simulink subsystem "ALU_64_BITS_05_SS"  (R2022a)
settings: Solver=VariableStepAuto  StartTime=0.0  StopTime=10.0  RelTol=1e-3
libraries: hdlBasic x1540
(part 1 of 7)
settings Model: Creator=sebas  LastModifiedBy=viktor

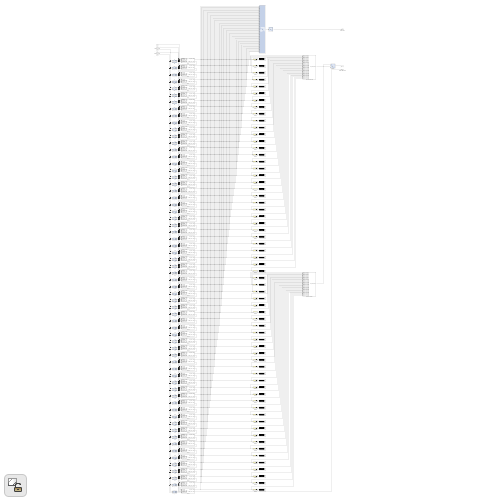
[thumbnail: Simulink's stored preview of the top-level diagram]
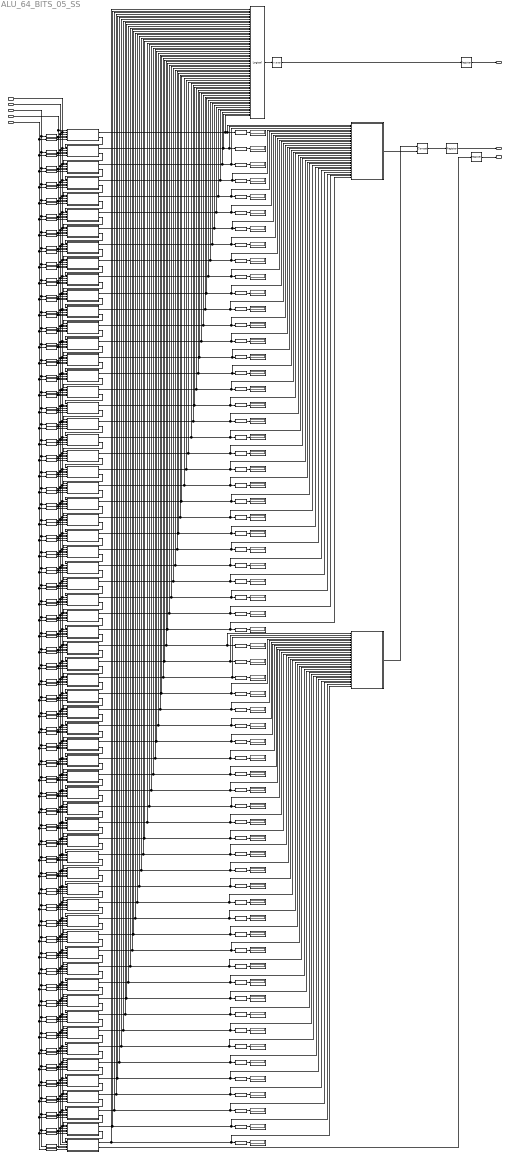
== system ALU_64_BITS_05_SS ==
  OPERATION (2 BIT) : Inport
  A_INVERT (1 BIT) : Inport  Port=2
  A_INPUT (64 BIT) : Inport  Port=3
  B_INVERT (1 BIT) : Inport  Port=4
  B_INPUT (64 BIT) : Inport  Port=5
  ALU_0 : Subsystem
  ALU_1 : Subsystem
  ALU_10 : Subsystem
  ALU_11 : Subsystem
  ALU_12 : Subsystem
  ALU_13 : Subsystem
  ALU_14 : Subsystem
  ALU_15 : Subsystem
  ALU_16 : Subsystem
  ALU_17 : Subsystem
  ALU_18 : Subsystem
  ALU_19 : Subsystem
  ALU_2 : Subsystem
  ALU_20 : Subsystem
  ALU_21 : Subsystem
  ALU_22 : Subsystem
  ALU_23 : Subsystem
  ALU_24 : Subsystem
  ALU_25 : Subsystem
  ALU_26 : Subsystem
  ALU_27 : Subsystem
  ALU_28 : Subsystem
  ALU_29 : Subsystem
  ALU_3 : Subsystem
  ALU_30 : Subsystem
  ALU_31 : Subsystem
  ALU_32 : Subsystem
  ALU_33 : Subsystem
  ALU_34 : Subsystem
  ALU_35 : Subsystem
  ALU_36 : Subsystem
  ALU_37 : Subsystem
  ALU_38 : Subsystem
  ALU_39 : Subsystem
  ALU_4 : Subsystem
  ALU_40 : Subsystem
  ALU_41 : Subsystem
  ALU_42 : Subsystem
  ALU_43 : Subsystem
  ALU_44 : Subsystem
  ALU_45 : Subsystem
  ALU_46 : Subsystem
  ALU_47 : Subsystem
  ALU_48 : Subsystem
  ALU_49 : Subsystem
  ALU_5 : Subsystem
  ALU_50 : Subsystem
  ALU_51 : Subsystem
  ALU_52 : Subsystem
  ALU_53 : Subsystem
  ALU_54 : Subsystem
  ALU_55 : Subsystem
  ALU_56 : Subsystem
  ALU_57 : Subsystem
  ALU_58 : Subsystem
  ALU_59 : Subsystem
  ALU_6 : Subsystem
  ALU_60 : Subsystem
  ALU_61 : Subsystem
  ALU_62 : Subsystem
  ALU_63 : Subsystem
  ALU_7 : Subsystem
  ALU_8 : Subsystem
  ALU_9 : Subsystem
  ALU_OUT_32_BIT_00 : Subsystem
  ALU_OUT_32_BIT_1 : Subsystem
  A_0 : hdlBasic/Slice  nbits=1  boolean_output=off  mode=Lower Bit Location + Width  bit1=-3  base1=MSB of Input  bit0=0  base0=LSB of Input  XmcBlockStatus=1  maskContainerNames=group1  block_type=slice  block_config=sysgen:Slice_config
  A_1 : hdlBasic/Slice  nbits=1  boolean_output=off  mode=Lower Bit Location + Width  bit1=-3  base1=MSB of Input  bit0=1  base0=LSB of Input  XmcBlockStatus=1  maskContainerNames=group1  block_type=slice  block_config=sysgen:Slice_config
  A_10 : hdlBasic/Slice  nbits=1  boolean_output=off  mode=Lower Bit Location + Width  bit1=-3  base1=MSB of Input  bit0=10  base0=LSB of Input  XmcBlockStatus=1  maskContainerNames=group1  block_type=slice  block_config=sysgen:Slice_config
  A_11 : hdlBasic/Slice  nbits=1  boolean_output=off  mode=Lower Bit Location + Width  bit1=-3  base1=MSB of Input  bit0=11  base0=LSB of Input  XmcBlockStatus=1  maskContainerNames=group1  block_type=slice  block_config=sysgen:Slice_config
  A_12 : hdlBasic/Slice  nbits=1  boolean_output=off  mode=Lower Bit Location + Width  bit1=-3  base1=MSB of Input  bit0=12  base0=LSB of Input  XmcBlockStatus=1  maskContainerNames=group1  block_type=slice  block_config=sysgen:Slice_config
  A_13 : hdlBasic/Slice  nbits=1  boolean_output=off  mode=Lower Bit Location + Width  bit1=-3  base1=MSB of Input  bit0=13  base0=LSB of Input  XmcBlockStatus=1  maskContainerNames=group1  block_type=slice  block_config=sysgen:Slice_config
  A_14 : hdlBasic/Slice  nbits=1  boolean_output=off  mode=Lower Bit Location + Width  bit1=-3  base1=MSB of Input  bit0=14  base0=LSB of Input  XmcBlockStatus=1  maskContainerNames=group1  block_type=slice  block_config=sysgen:Slice_config
  A_15 : hdlBasic/Slice  nbits=1  boolean_output=off  mode=Lower Bit Location + Width  bit1=-3  base1=MSB of Input  bit0=15  base0=LSB of Input  XmcBlockStatus=1  maskContainerNames=group1  block_type=slice  block_config=sysgen:Slice_config
  A_16 : hdlBasic/Slice  nbits=1  boolean_output=off  mode=Lower Bit Location + Width  bit1=-3  base1=MSB of Input  bit0=16  base0=LSB of Input  XmcBlockStatus=1  maskContainerNames=group1  block_type=slice  block_config=sysgen:Slice_config
  A_17 : hdlBasic/Slice  nbits=1  boolean_output=off  mode=Lower Bit Location + Width  bit1=-3  base1=MSB of Input  bit0=17  base0=LSB of Input  XmcBlockStatus=1  maskContainerNames=group1  block_type=slice  block_config=sysgen:Slice_config
  A_18 : hdlBasic/Slice  nbits=1  boolean_output=off  mode=Lower Bit Location + Width  bit1=-3  base1=MSB of Input  bit0=18  base0=LSB of Input  XmcBlockStatus=1  maskContainerNames=group1  block_type=slice  block_config=sysgen:Slice_config
  A_19 : hdlBasic/Slice  nbits=1  boolean_output=off  mode=Lower Bit Location + Width  bit1=-3  base1=MSB of Input  bit0=19  base0=LSB of Input  XmcBlockStatus=1  maskContainerNames=group1  block_type=slice  block_config=sysgen:Slice_config
  A_2 : hdlBasic/Slice  nbits=1  boolean_output=off  mode=Lower Bit Location + Width  bit1=-3  base1=MSB of Input  bit0=2  base0=LSB of Input  XmcBlockStatus=1  maskContainerNames=group1  block_type=slice  block_config=sysgen:Slice_config
  A_20 : hdlBasic/Slice  nbits=1  boolean_output=off  mode=Lower Bit Location + Width  bit1=-3  base1=MSB of Input  bit0=20  base0=LSB of Input  XmcBlockStatus=1  maskContainerNames=group1  block_type=slice  block_config=sysgen:Slice_config
  A_21 : hdlBasic/Slice  nbits=1  boolean_output=off  mode=Lower Bit Location + Width  bit1=-3  base1=MSB of Input  bit0=21  base0=LSB of Input  XmcBlockStatus=1  maskContainerNames=group1  block_type=slice  block_config=sysgen:Slice_config
  A_22 : hdlBasic/Slice  nbits=1  boolean_output=off  mode=Lower Bit Location + Width  bit1=-3  base1=MSB of Input  bit0=22  base0=LSB of Input  XmcBlockStatus=1  maskContainerNames=group1  block_type=slice  block_config=sysgen:Slice_config
  A_23 : hdlBasic/Slice  nbits=1  boolean_output=off  mode=Lower Bit Location + Width  bit1=-3  base1=MSB of Input  bit0=23  base0=LSB of Input  XmcBlockStatus=1  maskContainerNames=group1  block_type=slice  block_config=sysgen:Slice_config
  A_24 : hdlBasic/Slice  nbits=1  boolean_output=off  mode=Lower Bit Location + Width  bit1=-3  base1=MSB of Input  bit0=24  base0=LSB of Input  XmcBlockStatus=1  maskContainerNames=group1  block_type=slice  block_config=sysgen:Slice_config
  A_25 : hdlBasic/Slice  nbits=1  boolean_output=off  mode=Lower Bit Location + Width  bit1=-3  base1=MSB of Input  bit0=25  base0=LSB of Input  XmcBlockStatus=1  maskContainerNames=group1  block_type=slice  block_config=sysgen:Slice_config
  A_26 : hdlBasic/Slice  nbits=1  boolean_output=off  mode=Lower Bit Location + Width  bit1=-3  base1=MSB of Input  bit0=26  base0=LSB of Input  XmcBlockStatus=1  maskContainerNames=group1  block_type=slice  block_config=sysgen:Slice_config
  A_27 : hdlBasic/Slice  nbits=1  boolean_output=off  mode=Lower Bit Location + Width  bit1=-3  base1=MSB of Input  bit0=27  base0=LSB of Input  XmcBlockStatus=1  maskContainerNames=group1  block_type=slice  block_config=sysgen:Slice_config
  A_28 : hdlBasic/Slice  nbits=1  boolean_output=off  mode=Lower Bit Location + Width  bit1=-3  base1=MSB of Input  bit0=28  base0=LSB of Input  XmcBlockStatus=1  maskContainerNames=group1  block_type=slice  block_config=sysgen:Slice_config
  A_29 : hdlBasic/Slice  nbits=1  boolean_output=off  mode=Lower Bit Location + Width  bit1=-3  base1=MSB of Input  bit0=29  base0=LSB of Input  XmcBlockStatus=1  maskContainerNames=group1  block_type=slice  block_config=sysgen:Slice_config
  A_3 : hdlBasic/Slice  nbits=1  boolean_output=off  mode=Lower Bit Location + Width  bit1=-3  base1=MSB of Input  bit0=3  base0=LSB of Input  XmcBlockStatus=1  maskContainerNames=group1  block_type=slice  block_config=sysgen:Slice_config
  A_30 : hdlBasic/Slice  nbits=1  boolean_output=off  mode=Lower Bit Location + Width  bit1=-3  base1=MSB of Input  bit0=30  base0=LSB of Input  XmcBlockStatus=1  maskContainerNames=group1  block_type=slice  block_config=sysgen:Slice_config
  A_31 : hdlBasic/Slice  nbits=1  boolean_output=off  mode=Lower Bit Location + Width  bit1=-3  base1=MSB of Input  bit0=31  base0=LSB of Input  XmcBlockStatus=1  maskContainerNames=group1  block_type=slice  block_config=sysgen:Slice_config
  A_32 : hdlBasic/Slice  nbits=1  boolean_output=off  mode=Lower Bit Location + Width  bit1=-3  base1=MSB of Input  bit0=32  base0=LSB of Input  XmcBlockStatus=1  maskContainerNames=group1  block_type=slice  block_config=sysgen:Slice_config
  A_33 : hdlBasic/Slice  nbits=1  boolean_output=off  mode=Lower Bit Location + Width  bit1=-3  base1=MSB of Input  bit0=33  base0=LSB of Input  XmcBlockStatus=1  maskContainerNames=group1  block_type=slice  block_config=sysgen:Slice_config
  A_34 : hdlBasic/Slice  nbits=1  boolean_output=off  mode=Lower Bit Location + Width  bit1=-3  base1=MSB of Input  bit0=34  base0=LSB of Input  XmcBlockStatus=1  maskContainerNames=group1  block_type=slice  block_config=sysgen:Slice_config
  A_35 : hdlBasic/Slice  nbits=1  boolean_output=off  mode=Lower Bit Location + Width  bit1=-3  base1=MSB of Input  bit0=35  base0=LSB of Input  XmcBlockStatus=1  maskContainerNames=group1  block_type=slice  block_config=sysgen:Slice_config
  A_36 : hdlBasic/Slice  nbits=1  boolean_output=off  mode=Lower Bit Location + Width  bit1=-3  base1=MSB of Input  bit0=36  base0=LSB of Input  XmcBlockStatus=1  maskContainerNames=group1  block_type=slice  block_config=sysgen:Slice_config
  A_37 : hdlBasic/Slice  nbits=1  boolean_output=off  mode=Lower Bit Location + Width  bit1=-3  base1=MSB of Input  bit0=37  base0=LSB of Input  XmcBlockStatus=1  maskContainerNames=group1  block_type=slice  block_config=sysgen:Slice_config
  A_38 : hdlBasic/Slice  nbits=1  boolean_output=off  mode=Lower Bit Location + Width  bit1=-3  base1=MSB of Input  bit0=38  base0=LSB of Input  XmcBlockStatus=1  maskContainerNames=group1  block_type=slice  block_config=sysgen:Slice_config
  A_39 : hdlBasic/Slice  nbits=1  boolean_output=off  mode=Lower Bit Location + Width  bit1=-3  base1=MSB of Input  bit0=39  base0=LSB of Input  XmcBlockStatus=1  maskContainerNames=group1  block_type=slice  block_config=sysgen:Slice_config
  A_4 : hdlBasic/Slice  nbits=1  boolean_output=off  mode=Lower Bit Location + Width  bit1=-3  base1=MSB of Input  bit0=4  base0=LSB of Input  XmcBlockStatus=1  maskContainerNames=group1  block_type=slice  block_config=sysgen:Slice_config
  A_40 : hdlBasic/Slice  nbits=1  boolean_output=off  mode=Lower Bit Location + Width  bit1=-3  base1=MSB of Input  bit0=40  base0=LSB of Input  XmcBlockStatus=1  maskContainerNames=group1  block_type=slice  block_config=sysgen:Slice_config
  A_41 : hdlBasic/Slice  nbits=1  boolean_output=off  mode=Lower Bit Location + Width  bit1=-3  base1=MSB of Input  bit0=41  base0=LSB of Input  XmcBlockStatus=1  maskContainerNames=group1  block_type=slice  block_config=sysgen:Slice_config
  A_42 : hdlBasic/Slice  nbits=1  boolean_output=off  mode=Lower Bit Location + Width  bit1=-3  base1=MSB of Input  bit0=42  base0=LSB of Input  XmcBlockStatus=1  maskContainerNames=group1  block_type=slice  block_config=sysgen:Slice_config
  A_43 : hdlBasic/Slice  nbits=1  boolean_output=off  mode=Lower Bit Location + Width  bit1=-3  base1=MSB of Input  bit0=43  base0=LSB of Input  XmcBlockStatus=1  maskContainerNames=group1  block_type=slice  block_config=sysgen:Slice_config
  A_44 : hdlBasic/Slice  nbits=1  boolean_output=off  mode=Lower Bit Location + Width  bit1=-3  base1=MSB of Input  bit0=44  base0=LSB of Input  XmcBlockStatus=1  maskContainerNames=group1  block_type=slice  block_config=sysgen:Slice_config
  A_45 : hdlBasic/Slice  nbits=1  boolean_output=off  mode=Lower Bit Location + Width  bit1=-3  base1=MSB of Input  bit0=45  base0=LSB of Input  XmcBlockStatus=1  maskContainerNames=group1  block_type=slice  block_config=sysgen:Slice_config
  A_46 : hdlBasic/Slice  nbits=1  boolean_output=off  mode=Lower Bit Location + Width  bit1=-3  base1=MSB of Input  bit0=46  base0=LSB of Input  XmcBlockStatus=1  maskContainerNames=group1  block_type=slice  block_config=sysgen:Slice_config
  A_47 : hdlBasic/Slice  nbits=1  boolean_output=off  mode=Lower Bit Location + Width  bit1=-3  base1=MSB of Input  bit0=47  base0=LSB of Input  XmcBlockStatus=1  maskContainerNames=group1  block_type=slice  block_config=sysgen:Slice_config
  A_48 : hdlBasic/Slice  nbits=1  boolean_output=off  mode=Lower Bit Location + Width  bit1=-3  base1=MSB of Input  bit0=48  base0=LSB of Input  XmcBlockStatus=1  maskContainerNames=group1  block_type=slice  block_config=sysgen:Slice_config
  A_49 : hdlBasic/Slice  nbits=1  boolean_output=off  mode=Lower Bit Location + Width  bit1=-3  base1=MSB of Input  bit0=49  base0=LSB of Input  XmcBlockStatus=1  maskContainerNames=group1  block_type=slice  block_config=sysgen:Slice_config
  A_5 : hdlBasic/Slice  nbits=1  boolean_output=off  mode=Lower Bit Location + Width  bit1=-3  base1=MSB of Input  bit0=5  base0=LSB of Input  XmcBlockStatus=1  maskContainerNames=group1  block_type=slice  block_config=sysgen:Slice_config
  A_50 : hdlBasic/Slice  nbits=1  boolean_output=off  mode=Lower Bit Location + Width  bit1=-3  base1=MSB of Input  bit0=50  base0=LSB of Input  XmcBlockStatus=1  maskContainerNames=group1  block_type=slice  block_config=sysgen:Slice_config
  A_51 : hdlBasic/Slice  nbits=1  boolean_output=off  mode=Lower Bit Location + Width  bit1=-3  base1=MSB of Input  bit0=51  base0=LSB of Input  XmcBlockStatus=1  maskContainerNames=group1  block_type=slice  block_config=sysgen:Slice_config
  A_52 : hdlBasic/Slice  nbits=1  boolean_output=off  mode=Lower Bit Location + Width  bit1=-3  base1=MSB of Input  bit0=52  base0=LSB of Input  XmcBlockStatus=1  maskContainerNames=group1  block_type=slice  block_config=sysgen:Slice_config
  A_53 : hdlBasic/Slice  nbits=1  boolean_output=off  mode=Lower Bit Location + Width  bit1=-3  base1=MSB of Input  bit0=53  base0=LSB of Input  XmcBlockStatus=1  maskContainerNames=group1  block_type=slice  block_config=sysgen:Slice_config
  A_54 : hdlBasic/Slice  nbits=1  boolean_output=off  mode=Lower Bit Location + Width  bit1=-3  base1=MSB of Input  bit0=54  base0=LSB of Input  XmcBlockStatus=1  maskContainerNames=group1  block_type=slice  block_config=sysgen:Slice_config
  A_55 : hdlBasic/Slice  nbits=1  boolean_output=off  mode=Lower Bit Location + Width  bit1=-3  base1=MSB of Input  bit0=55  base0=LSB of Input  XmcBlockStatus=1  maskContainerNames=group1  block_type=slice  block_config=sysgen:Slice_config
  A_56 : hdlBasic/Slice  nbits=1  boolean_output=off  mode=Lower Bit Location + Width  bit1=-3  base1=MSB of Input  bit0=56  base0=LSB of Input  XmcBlockStatus=1  maskContainerNames=group1  block_type=slice  block_config=sysgen:Slice_config
  A_57 : hdlBasic/Slice  nbits=1  boolean_output=off  mode=Lower Bit Location + Width  bit1=-3  base1=MSB of Input  bit0=57  base0=LSB of Input  XmcBlockStatus=1  maskContainerNames=group1  block_type=slice  block_config=sysgen:Slice_config
  A_58 : hdlBasic/Slice  nbits=1  boolean_output=off  mode=Lower Bit Location + Width  bit1=-3  base1=MSB of Input  bit0=58  base0=LSB of Input  XmcBlockStatus=1  maskContainerNames=group1  block_type=slice  block_config=sysgen:Slice_config
  A_59 : hdlBasic/Slice  nbits=1  boolean_output=off  mode=Lower Bit Location + Width  bit1=-3  base1=MSB of Input  bit0=59  base0=LSB of Input  XmcBlockStatus=1  maskContainerNames=group1  block_type=slice  block_config=sysgen:Slice_config
  A_6 : hdlBasic/Slice  nbits=1  boolean_output=off  mode=Lower Bit Location + Width  bit1=-3  base1=MSB of Input  bit0=6  base0=LSB of Input  XmcBlockStatus=1  maskContainerNames=group1  block_type=slice  block_config=sysgen:Slice_config
  A_60 : hdlBasic/Slice  nbits=1  boolean_output=off  mode=Lower Bit Location + Width  bit1=-3  base1=MSB of Input  bit0=60  base0=LSB of Input  XmcBlockStatus=1  maskContainerNames=group1  block_type=slice  block_config=sysgen:Slice_config
  A_61 : hdlBasic/Slice  nbits=1  boolean_output=off  mode=Lower Bit Location + Width  bit1=-3  base1=MSB of Input  bit0=61  base0=LSB of Input  XmcBlockStatus=1  maskContainerNames=group1  block_type=slice  block_config=sysgen:Slice_config
  A_62 : hdlBasic/Slice  nbits=1  boolean_output=off  mode=Lower Bit Location + Width  bit1=-3  base1=MSB of Input  bit0=62  base0=LSB of Input  XmcBlockStatus=1  maskContainerNames=group1  block_type=slice  block_config=sysgen:Slice_config
  A_63 : hdlBasic/Slice  nbits=1  boolean_output=off  mode=Lower Bit Location + Width  bit1=-3  base1=MSB of Input  bit0=63  base0=LSB of Input  XmcBlockStatus=1  maskContainerNames=group1  block_type=slice  block_config=sysgen:Slice_config
  A_7 : hdlBasic/Slice  nbits=1  boolean_output=off  mode=Lower Bit Location + Width  bit1=-3  base1=MSB of Input  bit0=7  base0=LSB of Input  XmcBlockStatus=1  maskContainerNames=group1  block_type=slice  block_config=sysgen:Slice_config
  A_8 : hdlBasic/Slice  nbits=1  boolean_output=off  mode=Lower Bit Location + Width  bit1=-3  base1=MSB of Input  bit0=8  base0=LSB of Input  XmcBlockStatus=1  maskContainerNames=group1  block_type=slice  block_config=sysgen:Slice_config
  A_9 : hdlBasic/Slice  nbits=1  boolean_output=off  mode=Lower Bit Location + Width  bit1=-3  base1=MSB of Input  bit0=9  base0=LSB of Input  XmcBlockStatus=1  maskContainerNames=group1  block_type=slice  block_config=sysgen:Slice_config
  B_0 : hdlBasic/Slice  nbits=1  boolean_output=off  mode=Lower Bit Location + Width  bit1=-3  base1=MSB of Input  bit0=0  base0=LSB of Input  XmcBlockStatus=1  maskContainerNames=group1  block_type=slice  block_config=sysgen:Slice_config
  B_1 : hdlBasic/Slice  nbits=1  boolean_output=off  mode=Lower Bit Location + Width  bit1=-3  base1=MSB of Input  bit0=1  base0=LSB of Input  XmcBlockStatus=1  maskContainerNames=group1  block_type=slice  block_config=sysgen:Slice_config
  B_10 : hdlBasic/Slice  nbits=1  boolean_output=off  mode=Lower Bit Location + Width  bit1=-3  base1=MSB of Input  bit0=10  base0=LSB of Input  XmcBlockStatus=1  maskContainerNames=group1  block_type=slice  block_config=sysgen:Slice_config
  B_11 : hdlBasic/Slice  nbits=1  boolean_output=off  mode=Lower Bit Location + Width  bit1=-3  base1=MSB of Input  bit0=11  base0=LSB of Input  XmcBlockStatus=1  maskContainerNames=group1  block_type=slice  block_config=sysgen:Slice_config
  B_12 : hdlBasic/Slice  nbits=1  boolean_output=off  mode=Lower Bit Location + Width  bit1=-3  base1=MSB of Input  bit0=12  base0=LSB of Input  XmcBlockStatus=1  maskContainerNames=group1  block_type=slice  block_config=sysgen:Slice_config
  B_13 : hdlBasic/Slice  nbits=1  boolean_output=off  mode=Lower Bit Location + Width  bit1=-3  base1=MSB of Input  bit0=13  base0=LSB of Input  XmcBlockStatus=1  maskContainerNames=group1  block_type=slice  block_config=sysgen:Slice_config
  B_14 : hdlBasic/Slice  nbits=1  boolean_output=off  mode=Lower Bit Location + Width  bit1=-3  base1=MSB of Input  bit0=14  base0=LSB of Input  XmcBlockStatus=1  maskContainerNames=group1  block_type=slice  block_config=sysgen:Slice_config
  B_15 : hdlBasic/Slice  nbits=1  boolean_output=off  mode=Lower Bit Location + Width  bit1=-3  base1=MSB of Input  bit0=15  base0=LSB of Input  XmcBlockStatus=1  maskContainerNames=group1  block_type=slice  block_config=sysgen:Slice_config
  B_16 : hdlBasic/Slice  nbits=1  boolean_output=off  mode=Lower Bit Location + Width  bit1=-3  base1=MSB of Input  bit0=16  base0=LSB of Input  XmcBlockStatus=1  maskContainerNames=group1  block_type=slice  block_config=sysgen:Slice_config
  B_17 : hdlBasic/Slice  nbits=1  boolean_output=off  mode=Lower Bit Location + Width  bit1=-3  base1=MSB of Input  bit0=17  base0=LSB of Input  XmcBlockStatus=1  maskContainerNames=group1  block_type=slice  block_config=sysgen:Slice_config
  B_18 : hdlBasic/Slice  nbits=1  boolean_output=off  mode=Lower Bit Location + Width  bit1=-3  base1=MSB of Input  bit0=18  base0=LSB of Input  XmcBlockStatus=1  maskContainerNames=group1  block_type=slice  block_config=sysgen:Slice_config
  B_19 : hdlBasic/Slice  nbits=1  boolean_output=off  mode=Lower Bit Location + Width  bit1=-3  base1=MSB of Input  bit0=19  base0=LSB of Input  XmcBlockStatus=1  maskContainerNames=group1  block_type=slice  block_config=sysgen:Slice_config
  B_2 : hdlBasic/Slice  nbits=1  boolean_output=off  mode=Lower Bit Location + Width  bit1=-3  base1=MSB of Input  bit0=2  base0=LSB of Input  XmcBlockStatus=1  maskContainerNames=group1  block_type=slice  block_config=sysgen:Slice_config
  B_20 : hdlBasic/Slice  nbits=1  boolean_output=off  mode=Lower Bit Location + Width  bit1=-3  base1=MSB of Input  bit0=20  base0=LSB of Input  XmcBlockStatus=1  maskContainerNames=group1  block_type=slice  block_config=sysgen:Slice_config
  B_21 : hdlBasic/Slice  nbits=1  boolean_output=off  mode=Lower Bit Location + Width  bit1=-3  base1=MSB of Input  bit0=21  base0=LSB of Input  XmcBlockStatus=1  maskContainerNames=group1  block_type=slice  block_config=sysgen:Slice_config
  B_22 : hdlBasic/Slice  nbits=1  boolean_output=off  mode=Lower Bit Location + Width  bit1=-3  base1=MSB of Input  bit0=22  base0=LSB of Input  XmcBlockStatus=1  maskContainerNames=group1  block_type=slice  block_config=sysgen:Slice_config
  B_23 : hdlBasic/Slice  nbits=1  boolean_output=off  mode=Lower Bit Location + Width  bit1=-3  base1=MSB of Input  bit0=23  base0=LSB of Input  XmcBlockStatus=1  maskContainerNames=group1  block_type=slice  block_config=sysgen:Slice_config
  B_24 : hdlBasic/Slice  nbits=1  boolean_output=off  mode=Lower Bit Location + Width  bit1=-3  base1=MSB of Input  bit0=24  base0=LSB of Input  XmcBlockStatus=1  maskContainerNames=group1  block_type=slice  block_config=sysgen:Slice_config
  B_25 : hdlBasic/Slice  nbits=1  boolean_output=off  mode=Lower Bit Location + Width  bit1=-3  base1=MSB of Input  bit0=25  base0=LSB of Input  XmcBlockStatus=1  maskContainerNames=group1  block_type=slice  block_config=sysgen:Slice_config
  B_26 : hdlBasic/Slice  nbits=1  boolean_output=off  mode=Lower Bit Location + Width  bit1=-3  base1=MSB of Input  bit0=26  base0=LSB of Input  XmcBlockStatus=1  maskContainerNames=group1  block_type=slice  block_config=sysgen:Slice_config
  B_27 : hdlBasic/Slice  nbits=1  boolean_output=off  mode=Lower Bit Location + Width  bit1=-3  base1=MSB of Input  bit0=27  base0=LSB of Input  XmcBlockStatus=1  maskContainerNames=group1  block_type=slice  block_config=sysgen:Slice_config
  B_28 : hdlBasic/Slice  nbits=1  boolean_output=off  mode=Lower Bit Location + Width  bit1=-3  base1=MSB of Input  bit0=28  base0=LSB of Input  XmcBlockStatus=1  maskContainerNames=group1  block_type=slice  block_config=sysgen:Slice_config
  B_29 : hdlBasic/Slice  nbits=1  boolean_output=off  mode=Lower Bit Location + Width  bit1=-3  base1=MSB of Input  bit0=29  base0=LSB of Input  XmcBlockStatus=1  maskContainerNames=group1  block_type=slice  block_config=sysgen:Slice_config
  B_3 : hdlBasic/Slice  nbits=1  boolean_output=off  mode=Lower Bit Location + Width  bit1=-3  base1=MSB of Input  bit0=3  base0=LSB of Input  XmcBlockStatus=1  maskContainerNames=group1  block_type=slice  block_config=sysgen:Slice_config
  B_30 : hdlBasic/Slice  nbits=1  boolean_output=off  mode=Lower Bit Location + Width  bit1=-3  base1=MSB of Input  bit0=30  base0=LSB of Input  XmcBlockStatus=1  maskContainerNames=group1  block_type=slice  block_config=sysgen:Slice_config
  B_31 : hdlBasic/Slice  nbits=1  boolean_output=off  mode=Lower Bit Location + Width  bit1=-3  base1=MSB of Input  bit0=31  base0=LSB of Input  XmcBlockStatus=1  maskContainerNames=group1  block_type=slice  block_config=sysgen:Slice_config
  B_32 : hdlBasic/Slice  nbits=1  boolean_output=off  mode=Lower Bit Location + Width  bit1=-3  base1=MSB of Input  bit0=32  base0=LSB of Input  XmcBlockStatus=1  maskContainerNames=group1  block_type=slice  block_config=sysgen:Slice_config
  B_33 : hdlBasic/Slice  nbits=1  boolean_output=off  mode=Lower Bit Location + Width  bit1=-3  base1=MSB of Input  bit0=33  base0=LSB of Input  XmcBlockStatus=1  maskContainerNames=group1  block_type=slice  block_config=sysgen:Slice_config
  B_34 : hdlBasic/Slice  nbits=1  boolean_output=off  mode=Lower Bit Location + Width  bit1=-3  base1=MSB of Input  bit0=34  base0=LSB of Input  XmcBlockStatus=1  maskContainerNames=group1  block_type=slice  block_config=sysgen:Slice_config
  B_35 : hdlBasic/Slice  nbits=1  boolean_output=off  mode=Lower Bit Location + Width  bit1=-3  base1=MSB of Input  bit0=35  base0=LSB of Input  XmcBlockStatus=1  maskContainerNames=group1  block_type=slice  block_config=sysgen:Slice_config
  B_36 : hdlBasic/Slice  nbits=1  boolean_output=off  mode=Lower Bit Location + Width  bit1=-3  base1=MSB of Input  bit0=36  base0=LSB of Input  XmcBlockStatus=1  maskContainerNames=group1  block_type=slice  block_config=sysgen:Slice_config
  B_37 : hdlBasic/Slice  nbits=1  boolean_output=off  mode=Lower Bit Location + Width  bit1=-3  base1=MSB of Input  bit0=37  base0=LSB of Input  XmcBlockStatus=1  maskContainerNames=group1  block_type=slice  block_config=sysgen:Slice_config
  B_38 : hdlBasic/Slice  nbits=1  boolean_output=off  mode=Lower Bit Location + Width  bit1=-3  base1=MSB of Input  bit0=38  base0=LSB of Input  XmcBlockStatus=1  maskContainerNames=group1  block_type=slice  block_config=sysgen:Slice_config
  B_39 : hdlBasic/Slice  nbits=1  boolean_output=off  mode=Lower Bit Location + Width  bit1=-3  base1=MSB of Input  bit0=39  base0=LSB of Input  XmcBlockStatus=1  maskContainerNames=group1  block_type=slice  block_config=sysgen:Slice_config
  B_4 : hdlBasic/Slice  nbits=1  boolean_output=off  mode=Lower Bit Location + Width  bit1=-3  base1=MSB of Input  bit0=4  base0=LSB of Input  XmcBlockStatus=1  maskContainerNames=group1  block_type=slice  block_config=sysgen:Slice_config
  B_40 : hdlBasic/Slice  nbits=1  boolean_output=off  mode=Lower Bit Location + Width  bit1=-3  base1=MSB of Input  bit0=40  base0=LSB of Input  XmcBlockStatus=1  maskContainerNames=group1  block_type=slice  block_config=sysgen:Slice_config
  B_41 : hdlBasic/Slice  nbits=1  boolean_output=off  mode=Lower Bit Location + Width  bit1=-3  base1=MSB of Input  bit0=41  base0=LSB of Input  XmcBlockStatus=1  maskContainerNames=group1  block_type=slice  block_config=sysgen:Slice_config
  B_42 : hdlBasic/Slice  nbits=1  boolean_output=off  mode=Lower Bit Location + Width  bit1=-3  base1=MSB of Input  bit0=42  base0=LSB of Input  XmcBlockStatus=1  maskContainerNames=group1  block_type=slice  block_config=sysgen:Slice_config
  B_43 : hdlBasic/Slice  nbits=1  boolean_output=off  mode=Lower Bit Location + Width  bit1=-3  base1=MSB of Input  bit0=43  base0=LSB of Input  XmcBlockStatus=1  maskContainerNames=group1  block_type=slice  block_config=sysgen:Slice_config
  B_44 : hdlBasic/Slice  nbits=1  boolean_output=off  mode=Lower Bit Location + Width  bit1=-3  base1=MSB of Input  bit0=44  base0=LSB of Input  XmcBlockStatus=1  maskContainerNames=group1  block_type=slice  block_config=sysgen:Slice_config
  B_45 : hdlBasic/Slice  nbits=1  boolean_output=off  mode=Lower Bit Location + Width  bit1=-3  base1=MSB of Input  bit0=45  base0=LSB of Input  XmcBlockStatus=1  maskContainerNames=group1  block_type=slice  block_config=sysgen:Slice_config
  B_46 : hdlBasic/Slice  nbits=1  boolean_output=off  mode=Lower Bit Location + Width  bit1=-3  base1=MSB of Input  bit0=46  base0=LSB of Input  XmcBlockStatus=1  maskContainerNames=group1  block_type=slice  block_config=sysgen:Slice_config
  B_47 : hdlBasic/Slice  nbits=1  boolean_output=off  mode=Lower Bit Location + Width  bit1=-3  base1=MSB of Input  bit0=47  base0=LSB of Input  XmcBlockStatus=1  maskContainerNames=group1  block_type=slice  block_config=sysgen:Slice_config
  B_48 : hdlBasic/Slice  nbits=1  boolean_output=off  mode=Lower Bit Location + Width  bit1=-3  base1=MSB of Input  bit0=48  base0=LSB of Input  XmcBlockStatus=1  maskContainerNames=group1  block_type=slice  block_config=sysgen:Slice_config
  B_49 : hdlBasic/Slice  nbits=1  boolean_output=off  mode=Lower Bit Location + Width  bit1=-3  base1=MSB of Input  bit0=49  base0=LSB of Input  XmcBlockStatus=1  maskContainerNames=group1  block_type=slice  block_config=sysgen:Slice_config
  B_5 : hdlBasic/Slice  nbits=1  boolean_output=off  mode=Lower Bit Location + Width  bit1=-3  base1=MSB of Input  bit0=5  base0=LSB of Input  XmcBlockStatus=1  maskContainerNames=group1  block_type=slice  block_config=sysgen:Slice_config
  B_50 : hdlBasic/Slice  nbits=1  boolean_output=off  mode=Lower Bit Location + Width  bit1=-3  base1=MSB of Input  bit0=50  base0=LSB of Input  XmcBlockStatus=1  maskContainerNames=group1  block_type=slice  block_config=sysgen:Slice_config
  B_51 : hdlBasic/Slice  nbits=1  boolean_output=off  mode=Lower Bit Location + Width  bit1=-3  base1=MSB of Input  bit0=51  base0=LSB of Input  XmcBlockStatus=1  maskContainerNames=group1  block_type=slice  block_config=sysgen:Slice_config
  B_52 : hdlBasic/Slice  nbits=1  boolean_output=off  mode=Lower Bit Location + Width  bit1=-3  base1=MSB of Input  bit0=52  base0=LSB of Input  XmcBlockStatus=1  maskContainerNames=group1  block_type=slice  block_config=sysgen:Slice_config
  B_53 : hdlBasic/Slice  nbits=1  boolean_output=off  mode=Lower Bit Location + Width  bit1=-3  base1=MSB of Input  bit0=53  base0=LSB of Input  XmcBlockStatus=1  maskContainerNames=group1  block_type=slice  block_config=sysgen:Slice_config
  B_54 : hdlBasic/Slice  nbits=1  boolean_output=off  mode=Lower Bit Location + Width  bit1=-3  base1=MSB of Input  bit0=54  base0=LSB of Input  XmcBlockStatus=1  maskContainerNames=group1  block_type=slice  block_config=sysgen:Slice_config
  B_55 : hdlBasic/Slice  nbits=1  boolean_output=off  mode=Lower Bit Location + Width  bit1=-3  base1=MSB of Input  bit0=55  base0=LSB of Input  XmcBlockStatus=1  maskContainerNames=group1  block_type=slice  block_config=sysgen:Slice_config
  B_56 : hdlBasic/Slice  nbits=1  boolean_output=off  mode=Lower Bit Location + Width  bit1=-3  base1=MSB of Input  bit0=56  base0=LSB of Input  XmcBlockStatus=1  maskContainerNames=group1  block_type=slice  block_config=sysgen:Slice_config
  B_57 : hdlBasic/Slice  nbits=1  boolean_output=off  mode=Lower Bit Location + Width  bit1=-3  base1=MSB of Input  bit0=57  base0=LSB of Input  XmcBlockStatus=1  maskContainerNames=group1  block_type=slice  block_config=sysgen:Slice_config
  B_58 : hdlBasic/Slice  nbits=1  boolean_output=off  mode=Lower Bit Location + Width  bit1=-3  base1=MSB of Input  bit0=58  base0=LSB of Input  XmcBlockStatus=1  maskContainerNames=group1  block_type=slice  block_config=sysgen:Slice_config
  B_59 : hdlBasic/Slice  nbits=1  boolean_output=off  mode=Lower Bit Location + Width  bit1=-3  base1=MSB of Input  bit0=59  base0=LSB of Input  XmcBlockStatus=1  maskContainerNames=group1  block_type=slice  block_config=sysgen:Slice_config
  B_6 : hdlBasic/Slice  nbits=1  boolean_output=off  mode=Lower Bit Location + Width  bit1=-3  base1=MSB of Input  bit0=6  base0=LSB of Input  XmcBlockStatus=1  maskContainerNames=group1  block_type=slice  block_config=sysgen:Slice_config
  B_60 : hdlBasic/Slice  nbits=1  boolean_output=off  mode=Lower Bit Location + Width  bit1=-3  base1=MSB of Input  bit0=60  base0=LSB of Input  XmcBlockStatus=1  maskContainerNames=group1  block_type=slice  block_config=sysgen:Slice_config
  B_61 : hdlBasic/Slice  nbits=1  boolean_output=off  mode=Lower Bit Location + Width  bit1=-3  base1=MSB of Input  bit0=61  base0=LSB of Input  XmcBlockStatus=1  maskContainerNames=group1  block_type=slice  block_config=sysgen:Slice_config
  B_62 : hdlBasic/Slice  nbits=1  boolean_output=off  mode=Lower Bit Location + Width  bit1=-3  base1=MSB of Input  bit0=62  base0=LSB of Input  XmcBlockStatus=1  maskContainerNames=group1  block_type=slice  block_config=sysgen:Slice_config
  B_63 : hdlBasic/Slice  nbits=1  boolean_output=off  mode=Lower Bit Location + Width  bit1=-3  base1=MSB of Input  bit0=63  base0=LSB of Input  XmcBlockStatus=1  maskContainerNames=group1  block_type=slice  block_config=sysgen:Slice_config
  B_7 : hdlBasic/Slice  nbits=1  boolean_output=off  mode=Lower Bit Location + Width  bit1=-3  base1=MSB of Input  bit0=7  base0=LSB of Input  XmcBlockStatus=1  maskContainerNames=group1  block_type=slice  block_config=sysgen:Slice_config
  B_8 : hdlBasic/Slice  nbits=1  boolean_output=off  mode=Lower Bit Location + Width  bit1=-3  base1=MSB of Input  bit0=8  base0=LSB of Input  XmcBlockStatus=1  maskContainerNames=group1  block_type=slice  block_config=sysgen:Slice_config
  B_9 : hdlBasic/Slice  nbits=1  boolean_output=off  mode=Lower Bit Location + Width  bit1=-3  base1=MSB of Input  bit0=9  base0=LSB of Input  XmcBlockStatus=1  maskContainerNames=group1  block_type=slice  block_config=sysgen:Slice_config
  Concat1 : hdlBasic/Concat  num_inputs=2  XmcBlockStatus=1  maskContainerNames=group1  block_type=concat  block_config=sysgen:Concat_config
  Display{1..63,105} (64 alike) : Display
  Inverter : hdlBasic/Inverter  en=off  latency=0  XmcBlockStatus=1  maskContainerNames=group2  block_type=inv  block_config=sysgen:Inverter_config
  Register : hdlBasic/Register  init=0  rst=off  en=off  XmcBlockStatus=1  maskContainerNames=tabcontainer1  block_type=register  block_config=sysgen:Register_config
  Register1 : hdlBasic/Register  init=0  rst=off  en=off  XmcBlockStatus=1  maskContainerNames=tabcontainer1  block_type=register  block_config=sysgen:Register_config
  Register2 : hdlBasic/Register  init=0  rst=off  en=off  XmcBlockStatus=1  maskContainerNames=tabcontainer1  block_type=register  block_config=sysgen:Register_config
  Result{1..63,101} (64 alike) : hdlBasic/Gateway Out  inherit_from_input=off  hdl_port=on  rows=1  columns=1  UseAsDAC=off  DACChannel='1'  interface=None  automatic_assignment=on  address_offset=hex2dec('00')  intf_name=''  intf_description=''  timing_constraint=None  locs_specified=off  LOCs={}  io_standard={}  XmcBlockStatus=1  maskContainerNames=group4  block_type=gatewayout  block_config=sysgen:gateway_out_config  block_width_w=590  block_height_w=620  block_width=620  block_height=750
  ZERO : hdlBasic/Logical  logical_function=OR  inputs=64  en=off  latency=0  precision=User Defined  arith_type=Boolean  n_bits=1  bin_pt=0  align_bp=on  overflow=[]  quantization=[]  XmcBlockStatus=1  maskContainerNames=tabcontainer1  block_type=logical  block_config=sysgen:Logical_config
  ALU_OUT (64 BIT) : Outport
  CARRY_OUT (1 BIT) : Outport  Port=2
  ZERO (1 BIT) : Outport  Port=3
  wires:
  ALU_52/2(CARRY_OUT (1 BIT)) -> ALU_53/1(CARRY_IN (1 BIT))
  ALU_27/1(ALU_OUT (1 BIT)) -> Result26/1, ALU_OUT_32_BIT_00/28(ALU_OUT_27 (1 BIT)), ZERO/37
  A_INVERT (1 BIT)/1 -> ALU_0/3(A_INVERT (1 BIT)), ALU_1/3(A_INVERT (1 BIT)), ALU_2/3(A_INVERT (1 BIT)), ALU_3/3(A_INVERT (1 BIT)), ALU_4/3(A_INVERT (1 BIT)), ALU_5/3(A_INVERT (1 BIT)), ALU_6/3(A_INVERT (1 BIT)), ALU_7/3(A_INVERT (1 BIT)), ALU_8/3(A_INVERT (1 BIT)), ALU_9/3(A_INVERT (1 BIT)), ALU_10/3(A_INVERT (1 BIT)), ALU_11/3(A_INVERT (1 BIT)), ALU_12/3(A_INVERT (1 BIT)), ALU_13/3(A_INVERT (1 BIT)), ALU_14/3(A_INVERT (1 BIT)), ALU_15/3(A_INVERT (1 BIT)), ALU_16/3(A_INVERT (1 BIT)), ALU_17/3(A_INVERT (1 BIT)), ALU_18/3(A_INVERT (1 BIT)), ALU_19/3(A_INVERT (1 BIT)), ALU_20/3(A_INVERT (1 BIT)), ALU_21/3(A_INVERT (1 BIT)), ALU_22/3(A_INVERT (1 BIT)), ALU_23/3(A_INVERT (1 BIT)), ALU_24/3(A_INVERT (1 BIT)), ALU_25/3(A_INVERT (1 BIT)), ALU_26/3(A_INVERT (1 BIT)), ALU_27/3(A_INVERT (1 BIT)), ALU_28/3(A_INVERT (1 BIT)), ALU_29/3(A_INVERT (1 BIT)), ALU_30/3(A_INVERT (1 BIT)), ALU_31/3(A_INVERT (1 BIT)), ALU_32/3(A_INVERT (1 BIT)), ALU_33/3(A_INVERT (1 BIT)), ALU_34/3(A_INVERT (1 BIT)), ALU_35/3(A_INVERT (1 BIT)), ALU_36/3(A_INVERT (1 BIT)), ALU_37/3(A_INVERT (1 BIT)), ALU_38/3(A_INVERT (1 BIT)), ALU_39/3(A_INVERT (1 BIT)), ALU_40/3(A_INVERT (1 BIT)), ALU_41/3(A_INVERT (1 BIT)), ALU_42/3(A_INVERT (1 BIT)), ALU_43/3(A_INVERT (1 BIT)), ALU_44/3(A_INVERT (1 BIT)), ALU_45/3(A_INVERT (1 BIT)), ALU_46/3(A_INVERT (1 BIT)), ALU_47/3(A_INVERT (1 BIT)), ALU_48/3(A_INVERT (1 BIT)), ALU_49/3(A_INVERT (1 BIT)), ALU_50/3(A_INVERT (1 BIT)), ALU_51/3(A_INVERT (1 BIT)), ALU_52/3(A_INVERT (1 BIT)), ALU_53/3(A_INVERT (1 BIT)), ALU_54/3(A_INVERT (1 BIT)), ALU_55/3(A_INVERT (1 BIT)), ALU_56/3(A_INVERT (1 BIT)), ALU_57/3(A_INVERT (1 BIT)), ALU_58/3(A_INVERT (1 BIT)), ALU_59/3(A_INVERT (1 BIT)), ALU_61/3(A_INVERT (1 BIT)), ALU_63/3(A_INVERT (1 BIT)), ALU_62/3(A_INVERT (1 BIT)), ALU_60/3(A_INVERT (1 BIT))
  B_17/1 -> ALU_17/6(B_INPUT (1 BIT))
  ALU_17/1(ALU_OUT (1 BIT)) -> Result16/1, ALU_OUT_32_BIT_00/18(ALU_OUT_17 (1 BIT)), ZERO/47
  ALU_59/2(CARRY_OUT (1 BIT)) -> ALU_60/1(CARRY_IN (1 BIT))
  B_42/1 -> ALU_42/6(B_INPUT (1 BIT))
  Result58/1 -> Display58/1
  A_33/1 -> ALU_33/4(A_INPUT (1 BIT))
  ALU_60/1(ALU_OUT (1 BIT)) -> Result61/1, ALU_OUT_32_BIT_1/29(ALU_OUT_28 (1 BIT)), ZERO/4
  ALU_15/1(ALU_OUT (1 BIT)) -> Result14/1, ALU_OUT_32_BIT_00/16(ALU_OUT_15 (1 BIT)), ZERO/49
  Result5/1 -> Display5/1
  ALU_14/1(ALU_OUT (1 BIT)) -> Result15/1, ALU_OUT_32_BIT_00/15(ALU_OUT_14 (1 BIT)), ZERO/50
  B_INPUT (64 BIT)/1 -> B_0/1, B_2/1, B_3/1, B_4/1, B_5/1, B_6/1, B_7/1, B_8/1, B_9/1, B_10/1, B_11/1, B_12/1, B_13/1, B_15/1, B_16/1, B_17/1, B_18/1, B_19/1, B_20/1, B_21/1, B_22/1, B_23/1, B_24/1, B_25/1, B_26/1, B_27/1, B_28/1, B_29/1, B_30/1, B_31/1, B_32/1, B_33/1, B_34/1, B_35/1, B_36/1, B_37/1, B_38/1, B_39/1, B_40/1, B_41/1, B_42/1, B_43/1, B_44/1, B_46/1, B_47/1, B_48/1, B_49/1, B_50/1, B_51/1, B_52/1, B_53/1, B_54/1, B_55/1, B_56/1, B_57/1, B_58/1, B_59/1, B_60/1, B_61/1, B_62/1, B_63/1, B_45/1, B_14/1, B_1/1
  ALU_54/1(ALU_OUT (1 BIT)) -> Result55/1, ALU_OUT_32_BIT_1/23(ALU_OUT_22 (1 BIT)), ZERO/10
  ALU_32/1(ALU_OUT (1 BIT)) -> ALU_OUT_32_BIT_1/1(ALU_OUT_0 (1 BIT)), Result33/1, ZERO/32
  B_18/1 -> ALU_18/6(B_INPUT (1 BIT))
  ALU_3/2(CARRY_OUT (1 BIT)) -> ALU_4/1(CARRY_IN (1 BIT))
  B_INVERT (1 BIT)/1 -> ALU_0/5(B_INVERT (1 BIT)), ALU_1/5(B_INVERT (1 BIT)), ALU_2/5(B_INVERT (1 BIT)), ALU_3/5(B_INVERT (1 BIT)), ALU_4/5(B_INVERT (1 BIT)), ALU_5/5(B_INVERT (1 BIT)), ALU_6/5(B_INVERT (1 BIT)), ALU_7/5(B_INVERT (1 BIT)), ALU_8/5(B_INVERT (1 BIT)), ALU_9/5(B_INVERT (1 BIT)), ALU_10/5(B_INVERT (1 BIT)), ALU_11/5(B_INVERT (1 BIT)), ALU_12/5(B_INVERT (1 BIT)), ALU_13/5(B_INVERT (1 BIT)), ALU_14/5(B_INVERT (1 BIT)), ALU_15/5(B_INVERT (1 BIT)), ALU_16/5(B_INVERT (1 BIT)), ALU_17/5(B_INVERT (1 BIT)), ALU_18/5(B_INVERT (1 BIT)), ALU_19/5(B_INVERT (1 BIT)), ALU_20/5(B_INVERT (1 BIT)), ALU_21/5(B_INVERT (1 BIT)), ALU_22/5(B_INVERT (1 BIT)), ALU_23/5(B_INVERT (1 BIT)), ALU_24/5(B_INVERT (1 BIT)), ALU_25/5(B_INVERT (1 BIT)), ALU_26/5(B_INVERT (1 BIT)), ALU_27/5(B_INVERT (1 BIT)), ALU_28/5(B_INVERT (1 BIT)), ALU_29/5(B_INVERT (1 BIT)), ALU_30/5(B_INVERT (1 BIT)), ALU_31/5(B_INVERT (1 BIT)), ALU_32/5(B_INVERT (1 BIT)), ALU_33/5(B_INVERT (1 BIT)), ALU_34/5(B_INVERT (1 BIT)), ALU_35/5(B_INVERT (1 BIT)), ALU_36/5(B_INVERT (1 BIT)), ALU_37/5(B_INVERT (1 BIT)), ALU_38/5(B_INVERT (1 BIT)), ALU_39/5(B_INVERT (1 BIT)), ALU_40/5(B_INVERT (1 BIT)), ALU_41/5(B_INVERT (1 BIT)), ALU_42/5(B_INVERT (1 BIT)), ALU_43/5(B_INVERT (1 BIT)), ALU_44/5(B_INVERT (1 BIT)), ALU_45/5(B_INVERT (1 BIT)), ALU_46/5(B_INVERT (1 BIT)), ALU_47/5(B_INVERT (1 BIT)), ALU_48/5(B_INVERT (1 BIT)), ALU_49/5(B_INVERT (1 BIT)), ALU_50/5(B_INVERT (1 BIT)), ALU_51/5(B_INVERT (1 BIT)), ALU_52/5(B_INVERT (1 BIT)), ALU_53/5(B_INVERT (1 BIT)), ALU_54/5(B_INVERT (1 BIT)), ALU_55/5(B_INVERT (1 BIT)), ALU_56/5(B_INVERT (1 BIT)), ALU_57/5(B_INVERT (1 BIT)), ALU_58/5(B_INVERT (1 BIT)), ALU_59/5(B_INVERT (1 BIT)), ALU_60/5(B_INVERT (1 BIT)), ALU_61/5(B_INVERT (1 BIT)), ALU_63/5(B_INVERT (1 BIT)), ALU_62/5(B_INVERT (1 BIT)), ALU_0/1(CARRY_IN (1 BIT))
  ALU_20/2(CARRY_OUT (1 BIT)) -> ALU_21/1(CARRY_IN (1 BIT))
  ALU_16/1(ALU_OUT (1 BIT)) -> Result17/1, ALU_OUT_32_BIT_00/17(ALU_OUT_16 (1 BIT)), ZERO/48
  A_INPUT (64 BIT)/1 -> A_0/1, A_1/1, A_2/1, A_3/1, A_4/1, A_5/1, A_6/1, A_7/1, A_8/1, A_9/1, A_10/1, A_11/1, A_12/1, A_13/1, A_14/1, A_15/1, A_16/1, A_17/1, A_18/1, A_19/1, A_20/1, A_21/1, A_22/1, A_23/1, A_24/1, A_25/1, A_26/1, A_27/1, A_28/1, A_29/1, A_30/1, A_31/1, A_32/1, A_33/1, A_34/1, A_35/1, A_36/1, A_37/1, A_38/1, A_39/1, A_40/1, A_41/1, A_42/1, A_43/1, A_44/1, A_45/1, A_46/1, A_47/1, A_48/1, A_49/1, A_50/1, A_51/1, A_52/1, A_53/1, A_54/1, A_55/1, A_56/1, A_57/1, A_58/1, A_59/1, A_60/1, A_61/1, A_62/1, A_63/1
  ALU_47/1(ALU_OUT (1 BIT)) -> Result46/1, ALU_OUT_32_BIT_1/16(ALU_OUT_15 (1 BIT)), ZERO/17
  ALU_53/1(ALU_OUT (1 BIT)) -> Result52/1, ALU_OUT_32_BIT_1/22(ALU_OUT_21 (1 BIT)), ZERO/11
  A_55/1 -> ALU_55/4(A_INPUT (1 BIT))
  Result13/1 -> Display13/1
  OPERATION (2 BIT)/1 -> ALU_0/2(OP (2 BIT)), ALU_1/2(OP (2 BIT)), ALU_2/2(OP (2 BIT)), ALU_3/2(OP (2 BIT)), ALU_4/2(OP (2 BIT)), ALU_5/2(OP (2 BIT)), ALU_6/2(OP (2 BIT)), ALU_7/2(OP (2 BIT)), ALU_8/2(OP (2 BIT)), ALU_9/2(OP (2 BIT)), ALU_10/2(OP (2 BIT)), ALU_11/2(OP (2 BIT)), ALU_12/2(OP (2 BIT)), ALU_13/2(OP (2 BIT)), ALU_14/2(OP (2 BIT)), ALU_15/2(OP (2 BIT)), ALU_16/2(OP (2 BIT)), ALU_17/2(OP (2 BIT)), ALU_18/2(OP (2 BIT)), ALU_19/2(OP (2 BIT)), ALU_20/2(OP (2 BIT)), ALU_21/2(OP (2 BIT)), ALU_22/2(OP (2 BIT)), ALU_23/2(OP (2 BIT)), ALU_24/2(OP (2 BIT)), ALU_25/2(OP (2 BIT)), ALU_26/2(OP (2 BIT)), ALU_27/2(OP (2 BIT)), ALU_28/2(OP (2 BIT)), ALU_29/2(OP (2 BIT)), ALU_30/2(OP (2 BIT)), ALU_31/2(OP (2 BIT)), ALU_32/2(OP (2 BIT)), ALU_33/2(OP (2 BIT)), ALU_34/2(OP (2 BIT)), ALU_35/2(OP (2 BIT)), ALU_36/2(OP (2 BIT)), ALU_37/2(OP (2 BIT)), ALU_38/2(OP (2 BIT)), ALU_39/2(OP (2 BIT)), ALU_40/2(OP (2 BIT)), ALU_41/2(OP (2 BIT)), ALU_42/2(OP (2 BIT)), ALU_43/2(OP (2 BIT)), ALU_44/2(OP (2 BIT)), ALU_45/2(OP (2 BIT)), ALU_46/2(OP (2 BIT)), ALU_47/2(OP (2 BIT)), ALU_48/2(OP (2 BIT)), ALU_49/2(OP (2 BIT)), ALU_50/2(OP (2 BIT)), ALU_51/2(OP (2 BIT)), ALU_52/2(OP (2 BIT)), ALU_53/2(OP (2 BIT)), ALU_54/2(OP (2 BIT)), ALU_55/2(OP (2 BIT)), ALU_56/2(OP (2 BIT)), ALU_57/2(OP (2 BIT)), ALU_58/2(OP (2 BIT)), ALU_59/2(OP (2 BIT)), ALU_60/2(OP (2 BIT)), ALU_61/2(OP (2 BIT)), ALU_62/2(OP (2 BIT)), ALU_63/2(OP (2 BIT))
  ALU_45/2(CARRY_OUT (1 BIT)) -> ALU_46/1(CARRY_IN (1 BIT))
  ALU_61/1(ALU_OUT (1 BIT)) -> Result60/1, ALU_OUT_32_BIT_1/30(ALU_OUT_29 (1 BIT)), ZERO/3
  A_8/1 -> ALU_8/4(A_INPUT (1 BIT))
  A_15/1 -> ALU_15/4(A_INPUT (1 BIT))
  B_49/1 -> ALU_49/6(B_INPUT (1 BIT))
  B_8/1 -> ALU_8/6(B_INPUT (1 BIT))
  A_10/1 -> ALU_10/4(A_INPUT (1 BIT))
  A_11/1 -> ALU_11/4(A_INPUT (1 BIT))
  ALU_52/1(ALU_OUT (1 BIT)) -> Result53/1, ALU_OUT_32_BIT_1/21(ALU_OUT_20 (1 BIT)), ZERO/12
  ALU_11/1(ALU_OUT (1 BIT)) -> Result10/1, ALU_OUT_32_BIT_00/12(ALU_OUT_11 (1 BIT)), ZERO/53
  Result49/1 -> Display49/1
  Result57/1 -> Display57/1
  ALU_19/1(ALU_OUT (1 BIT)) -> ALU_OUT_32_BIT_00/20(ALU_OUT_19 (1 BIT)), Result18/1, ZERO/45
  Result33/1 -> Display33/1
  ALU_10/1(ALU_OUT (1 BIT)) -> Result11/1, ALU_OUT_32_BIT_00/11(ALU_OUT_10 (1 BIT)), ZERO/54
  ALU_41/1(ALU_OUT (1 BIT)) -> Result40/1, ALU_OUT_32_BIT_1/10(ALU_OUT_9 (1 BIT)), ZERO/23
  ALU_4/2(CARRY_OUT (1 BIT)) -> ALU_5/1(CARRY_IN (1 BIT))
  A_47/1 -> ALU_47/4(A_INPUT (1 BIT))
  Result14/1 -> Display14/1
  ALU_24/1(ALU_OUT (1 BIT)) -> Result25/1, ALU_OUT_32_BIT_00/25(ALU_OUT_24 (1 BIT)), ZERO/40
  A_35/1 -> ALU_35/4(A_INPUT (1 BIT))
  ALU_6/1(ALU_OUT (1 BIT)) -> ZERO/58, Result7/1, ALU_OUT_32_BIT_00/7(ALU_OUT_6 (1 BIT))
  Result54/1 -> Display54/1
  A_30/1 -> ALU_30/4(A_INPUT (1 BIT))
  ALU_42/1(ALU_OUT (1 BIT)) -> ALU_OUT_32_BIT_1/11(ALU_OUT_10 (1 BIT)), Result43/1, ZERO/22
  ALU_46/2(CARRY_OUT (1 BIT)) -> ALU_47/1(CARRY_IN (1 BIT))
  ALU_51/2(CARRY_OUT (1 BIT)) -> ALU_52/1(CARRY_IN (1 BIT))
  ALU_46/1(ALU_OUT (1 BIT)) -> Result47/1, ALU_OUT_32_BIT_1/15(ALU_OUT_14 (1 BIT)), ZERO/18
  ALU_38/2(CARRY_OUT (1 BIT)) -> ALU_39/1(CARRY_IN (1 BIT))
  A_32/1 -> ALU_32/4(A_INPUT (1 BIT))
  ALU_21/1(ALU_OUT (1 BIT)) -> Result20/1, ALU_OUT_32_BIT_00/22(ALU_OUT_21 (1 BIT)), ZERO/43
  ALU_62/1(ALU_OUT (1 BIT)) -> Result63/1, ALU_OUT_32_BIT_1/31(ALU_OUT_30 (1 BIT)), ZERO/2
  A_0/1 -> ALU_0/4(A_INPUT (1 BIT))
  Result15/1 -> Display15/1
  ALU_40/2(CARRY_OUT (1 BIT)) -> ALU_41/1(CARRY_IN (1 BIT))
  Result23/1 -> Display23/1
  B_57/1 -> ALU_57/6(B_INPUT (1 BIT))
  Result4/1 -> Display4/1
  ALU_OUT_32_BIT_1/1(ALU_OUT (32 BIT)) -> Concat1/1
  B_2/1 -> ALU_2/6(B_INPUT (1 BIT))
  ALU_7/1(ALU_OUT (1 BIT)) -> Result6/1, ALU_OUT_32_BIT_00/8(ALU_OUT_7 (1 BIT)), ZERO/57
  ALU_49/2(CARRY_OUT (1 BIT)) -> ALU_50/1(CARRY_IN (1 BIT))
  ALU_28/2(CARRY_OUT (1 BIT)) -> ALU_29/1(CARRY_IN (1 BIT))
  ALU_38/1(ALU_OUT (1 BIT)) -> ALU_OUT_32_BIT_1/7(ALU_OUT_6 (1 BIT)), Result39/1, ZERO/26
  ALU_48/1(ALU_OUT (1 BIT)) -> Result49/1, ALU_OUT_32_BIT_1/17(ALU_OUT_16 (1 BIT)), ZERO/16
  ALU_22/1(ALU_OUT (1 BIT)) -> Result23/1, ALU_OUT_32_BIT_00/23(ALU_OUT_22 (1 BIT)), ZERO/42
  ALU_39/1(ALU_OUT (1 BIT)) -> ZERO/25, Result38/1, ALU_OUT_32_BIT_1/8(ALU_OUT_7 (1 BIT))
  ALU_33/1(ALU_OUT (1 BIT)) -> ALU_OUT_32_BIT_1/2(ALU_OUT_1 (1 BIT)), Result32/1, ZERO/31
  B_53/1 -> ALU_53/6(B_INPUT (1 BIT))
  Result12/1 -> Display12/1
  ALU_57/1(ALU_OUT (1 BIT)) -> Result56/1, ALU_OUT_32_BIT_1/26(ALU_OUT_25 (1 BIT)), ZERO/7
  ALU_13/1(ALU_OUT (1 BIT)) -> Result12/1, ALU_OUT_32_BIT_00/14(ALU_OUT_13 (1 BIT)), ZERO/51
  ALU_56/1(ALU_OUT (1 BIT)) -> Result57/1, ALU_OUT_32_BIT_1/25(ALU_OUT_24 (1 BIT)), ZERO/8
  B_56/1 -> ALU_56/6(B_INPUT (1 BIT))
  B_6/1 -> ALU_6/6(B_INPUT (1 BIT))
  Result20/1 -> Display20/1
  ALU_40/1(ALU_OUT (1 BIT)) -> ZERO/24, Result41/1, ALU_OUT_32_BIT_1/9(ALU_OUT_8 (1 BIT))
  ALU_58/1(ALU_OUT (1 BIT)) -> Result59/1, ALU_OUT_32_BIT_1/27(ALU_OUT_26 (1 BIT)), ZERO/6
  B_32/1 -> ALU_32/6(B_INPUT (1 BIT))
  ALU_60/2(CARRY_OUT (1 BIT)) -> ALU_61/1(CARRY_IN (1 BIT))
  ALU_23/2(CARRY_OUT (1 BIT)) -> ALU_24/1(CARRY_IN (1 BIT))
  ALU_28/1(ALU_OUT (1 BIT)) -> Result29/1, ALU_OUT_32_BIT_00/29(ALU_OUT_28 (1 BIT)), ZERO/36
  ALU_36/1(ALU_OUT (1 BIT)) -> Result37/1, ALU_OUT_32_BIT_1/5(ALU_OUT_4 (1 BIT)), ZERO/28
  A_19/1 -> ALU_19/4(A_INPUT (1 BIT))
  ALU_61/2(CARRY_OUT (1 BIT)) -> ALU_62/1(CARRY_IN (1 BIT))
  A_26/1 -> ALU_26/4(A_INPUT (1 BIT))
  ALU_11/2(CARRY_OUT (1 BIT)) -> ALU_12/1(CARRY_IN (1 BIT))
  ALU_49/1(ALU_OUT (1 BIT)) -> Result48/1, ALU_OUT_32_BIT_1/18(ALU_OUT_17 (1 BIT)), ZERO/15
  A_62/1 -> ALU_62/4(A_INPUT (1 BIT))
  ALU_9/1(ALU_OUT (1 BIT)) -> Result8/1, ALU_OUT_32_BIT_00/10(ALU_OUT_9 (1 BIT)), ZERO/55
  B_25/1 -> ALU_25/6(B_INPUT (1 BIT))
  ALU_25/1(ALU_OUT (1 BIT)) -> ZERO/39, Result24/1, ALU_OUT_32_BIT_00/26(ALU_OUT_25 (1 BIT))
  Result60/1 -> Display60/1
  A_58/1 -> ALU_58/4(A_INPUT (1 BIT))
  ALU_31/1(ALU_OUT (1 BIT)) -> Result30/1, ALU_OUT_32_BIT_00/32(ALU_OUT_31 (1 BIT)), ZERO/33
  ALU_63/1(ALU_OUT (1 BIT)) -> Result62/1, ALU_OUT_32_BIT_1/32(ALU_OUT_31 (1 BIT)), ZERO/1
  ALU_4/1(ALU_OUT (1 BIT)) -> Result5/1, ALU_OUT_32_BIT_00/5(ALU_OUT_4 (1 BIT)), ZERO/60
  Result17/1 -> Display17/1
  Result61/1 -> Display61/1
  ALU_33/2(CARRY_OUT (1 BIT)) -> ALU_34/1(CARRY_IN (1 BIT))
  Result62/1 -> Display62/1
  Result31/1 -> Display31/1
  ALU_34/1(ALU_OUT (1 BIT)) -> ZERO/30, Result35/1, ALU_OUT_32_BIT_1/3(ALU_OUT_2 (1 BIT))
  Result22/1 -> Display22/1
  B_52/1 -> ALU_52/6(B_INPUT (1 BIT))
  ZERO/1 -> Inverter/1
  A_12/1 -> ALU_12/4(A_INPUT (1 BIT))
  Concat1/1 -> Register1/1
  ALU_1/1(ALU_OUT (1 BIT)) -> ALU_OUT_32_BIT_00/2(ALU_OUT_1 (1 BIT)), Result1/1, ZERO/63
  B_31/1 -> ALU_31/6(B_INPUT (1 BIT))
  A_20/1 -> ALU_20/4(A_INPUT (1 BIT))
  A_45/1 -> ALU_45/4(A_INPUT (1 BIT))
  Result25/1 -> Display25/1
  ALU_26/1(ALU_OUT (1 BIT)) -> ZERO/38, Result27/1, ALU_OUT_32_BIT_00/27(ALU_OUT_26 (1 BIT))
  A_52/1 -> ALU_52/4(A_INPUT (1 BIT))
  ALU_15/2(CARRY_OUT (1 BIT)) -> ALU_16/1(CARRY_IN (1 BIT))
  ALU_47/2(CARRY_OUT (1 BIT)) -> ALU_48/1(CARRY_IN (1 BIT))
  B_20/1 -> ALU_20/6(B_INPUT (1 BIT))
  B_59/1 -> ALU_59/6(B_INPUT (1 BIT))
  ALU_56/2(CARRY_OUT (1 BIT)) -> ALU_57/1(CARRY_IN (1 BIT))
  ALU_35/1(ALU_OUT (1 BIT)) -> ZERO/29, Result34/1, ALU_OUT_32_BIT_1/4(ALU_OUT_3 (1 BIT))
  ALU_21/2(CARRY_OUT (1 BIT)) -> ALU_22/1(CARRY_IN (1 BIT))
  ALU_25/2(CARRY_OUT (1 BIT)) -> ALU_26/1(CARRY_IN (1 BIT))
  ALU_59/1(ALU_OUT (1 BIT)) -> Result58/1, ALU_OUT_32_BIT_1/28(ALU_OUT_27 (1 BIT)), ZERO/5
  B_4/1 -> ALU_4/6(B_INPUT (1 BIT))
  Result2/1 -> Display2/1
  A_23/1 -> ALU_23/4(A_INPUT (1 BIT))
  Result24/1 -> Display24/1
  B_54/1 -> ALU_54/6(B_INPUT (1 BIT))
  ALU_27/2(CARRY_OUT (1 BIT)) -> ALU_28/1(CARRY_IN (1 BIT))
  B_33/1 -> ALU_33/6(B_INPUT (1 BIT))
  Result7/1 -> Display7/1
  ALU_5/1(ALU_OUT (1 BIT)) -> Result4/1, ALU_OUT_32_BIT_00/6(ALU_OUT_5 (1 BIT)), ZERO/59
  ALU_6/2(CARRY_OUT (1 BIT)) -> ALU_7/1(CARRY_IN (1 BIT))
  A_6/1 -> ALU_6/4(A_INPUT (1 BIT))
  A_63/1 -> ALU_63/4(A_INPUT (1 BIT))
  Result59/1 -> Display59/1
  ALU_2/1(ALU_OUT (1 BIT)) -> ALU_OUT_32_BIT_00/3(ALU_OUT_2 (1 BIT)), Result3/1, ZERO/62
  Result6/1 -> Display6/1
  A_61/1 -> ALU_61/4(A_INPUT (1 BIT))
  ALU_3/1(ALU_OUT (1 BIT)) -> Result2/1, ALU_OUT_32_BIT_00/4(ALU_OUT_3 (1 BIT)), ZERO/61
  B_13/1 -> ALU_13/6(B_INPUT (1 BIT))
  Result34/1 -> Display34/1
  ALU_55/1(ALU_OUT (1 BIT)) -> Result54/1, ALU_OUT_32_BIT_1/24(ALU_OUT_23 (1 BIT)), ZERO/9
  B_46/1 -> ALU_46/6(B_INPUT (1 BIT))
  ALU_0/2(CARRY_OUT (1 BIT)) -> ALU_1/1(CARRY_IN (1 BIT))
  Result16/1 -> Display16/1
  Result35/1 -> Display35/1
  Inverter/1 -> Register/1
  B_21/1 -> ALU_21/6(B_INPUT (1 BIT))
  ALU_43/1(ALU_OUT (1 BIT)) -> Result42/1, ALU_OUT_32_BIT_1/12(ALU_OUT_11 (1 BIT)), ZERO/21
  B_44/1 -> ALU_44/6(B_INPUT (1 BIT))
  A_34/1 -> ALU_34/4(A_INPUT (1 BIT))
  Result44/1 -> Display44/1
  ALU_24/2(CARRY_OUT (1 BIT)) -> ALU_25/1(CARRY_IN (1 BIT))
  A_3/1 -> ALU_3/4(A_INPUT (1 BIT))
  B_50/1 -> ALU_50/6(B_INPUT (1 BIT))
  A_43/1 -> ALU_43/4(A_INPUT (1 BIT))
  A_37/1 -> ALU_37/4(A_INPUT (1 BIT))
  ALU_22/2(CARRY_OUT (1 BIT)) -> ALU_23/1(CARRY_IN (1 BIT))
  B_34/1 -> ALU_34/6(B_INPUT (1 BIT))
  A_16/1 -> ALU_16/4(A_INPUT (1 BIT))
  A_60/1 -> ALU_60/4(A_INPUT (1 BIT))
  Result8/1 -> Display8/1
  ALU_23/1(ALU_OUT (1 BIT)) -> Result22/1, ALU_OUT_32_BIT_00/24(ALU_OUT_23 (1 BIT)), ZERO/41
  A_9/1 -> ALU_9/4(A_INPUT (1 BIT))
  ALU_45/1(ALU_OUT (1 BIT)) -> ALU_OUT_32_BIT_1/14(ALU_OUT_13 (1 BIT)), Result44/1, ZERO/19
  ALU_5/2(CARRY_OUT (1 BIT)) -> ALU_6/1(CARRY_IN (1 BIT))
  ALU_1/2(CARRY_OUT (1 BIT)) -> ALU_2/1(CARRY_IN (1 BIT))
  A_54/1 -> ALU_54/4(A_INPUT (1 BIT))
  Result45/1 -> Display45/1
  B_14/1 -> ALU_14/6(B_INPUT (1 BIT))
  ALU_0/1(ALU_OUT (1 BIT)) -> ALU_OUT_32_BIT_00/1(ALU_OUT_0 (1 BIT)), Result101/1, ZERO/64
  Result101/1 -> Display105/1
  Result41/1 -> Display41/1
  ALU_12/1(ALU_OUT (1 BIT)) -> Result13/1, ALU_OUT_32_BIT_00/13(ALU_OUT_12 (1 BIT)), ZERO/52
  ALU_8/2(CARRY_OUT (1 BIT)) -> ALU_9/1(CARRY_IN (1 BIT))
  B_51/1 -> ALU_51/6(B_INPUT (1 BIT))
  A_27/1 -> ALU_27/4(A_INPUT (1 BIT))
  ALU_42/2(CARRY_OUT (1 BIT)) -> ALU_43/1(CARRY_IN (1 BIT))
  ALU_44/1(ALU_OUT (1 BIT)) -> Result45/1, ALU_OUT_32_BIT_1/13(ALU_OUT_12 (1 BIT)), ZERO/20
  B_1/1 -> ALU_1/6(B_INPUT (1 BIT))
  B_10/1 -> ALU_10/6(B_INPUT (1 BIT))
  Result50/1 -> Display50/1
  ALU_37/1(ALU_OUT (1 BIT)) -> Result36/1, ALU_OUT_32_BIT_1/6(ALU_OUT_5 (1 BIT)), ZERO/27
  A_17/1 -> ALU_17/4(A_INPUT (1 BIT))
  Result10/1 -> Display10/1
  B_48/1 -> ALU_48/6(B_INPUT (1 BIT))
  ALU_8/1(ALU_OUT (1 BIT)) -> Result9/1, ALU_OUT_32_BIT_00/9(ALU_OUT_8 (1 BIT)), ZERO/56
  B_43/1 -> ALU_43/6(B_INPUT (1 BIT))
  ALU_9/2(CARRY_OUT (1 BIT)) -> ALU_10/1(CARRY_IN (1 BIT))
  Result21/1 -> Display21/1
  Result63/1 -> Display63/1
  A_22/1 -> ALU_22/4(A_INPUT (1 BIT))
  Result9/1 -> Display9/1
  ALU_10/2(CARRY_OUT (1 BIT)) -> ALU_11/1(CARRY_IN (1 BIT))
  Result11/1 -> Display11/1
  ALU_13/2(CARRY_OUT (1 BIT)) -> ALU_14/1(CARRY_IN (1 BIT))
  ALU_44/2(CARRY_OUT (1 BIT)) -> ALU_45/1(CARRY_IN (1 BIT))
  Result36/1 -> Display36/1
  Result19/1 -> Display19/1
  ALU_30/2(CARRY_OUT (1 BIT)) -> ALU_31/1(CARRY_IN (1 BIT))
  ALU_18/2(CARRY_OUT (1 BIT)) -> ALU_19/1(CARRY_IN (1 BIT))
  Result43/1 -> Display43/1
  ALU_53/2(CARRY_OUT (1 BIT)) -> ALU_54/1(CARRY_IN (1 BIT))
  ALU_17/2(CARRY_OUT (1 BIT)) -> ALU_18/1(CARRY_IN (1 BIT))
  Result53/1 -> Display53/1
  ALU_31/2(CARRY_OUT (1 BIT)) -> ALU_32/1(CARRY_IN (1 BIT))
  ALU_16/2(CARRY_OUT (1 BIT)) -> ALU_17/1(CARRY_IN (1 BIT))
  B_61/1 -> ALU_61/6(B_INPUT (1 BIT))
  ALU_18/1(ALU_OUT (1 BIT)) -> Result19/1, ALU_OUT_32_BIT_00/19(ALU_OUT_18 (1 BIT)), ZERO/46
  ALU_50/2(CARRY_OUT (1 BIT)) -> ALU_51/1(CARRY_IN (1 BIT))
  Result18/1 -> Display18/1
  Result42/1 -> Display42/1
  Result1/1 -> Display1/1
  B_38/1 -> ALU_38/6(B_INPUT (1 BIT))
  Result26/1 -> Display26/1
  Result48/1 -> Display48/1
  A_48/1 -> ALU_48/4(A_INPUT (1 BIT))
  ALU_20/1(ALU_OUT (1 BIT)) -> Result21/1, ALU_OUT_32_BIT_00/21(ALU_OUT_20 (1 BIT)), ZERO/44
  B_55/1 -> ALU_55/6(B_INPUT (1 BIT))
  A_38/1 -> ALU_38/4(A_INPUT (1 BIT))
  ALU_12/2(CARRY_OUT (1 BIT)) -> ALU_13/1(CARRY_IN (1 BIT))
  B_29/1 -> ALU_29/6(B_INPUT (1 BIT))
  A_39/1 -> ALU_39/4(A_INPUT (1 BIT))
  A_40/1 -> ALU_40/4(A_INPUT (1 BIT))
  A_49/1 -> ALU_49/4(A_INPUT (1 BIT))
  ALU_29/1(ALU_OUT (1 BIT)) -> ZERO/35, Result28/1, ALU_OUT_32_BIT_00/30(ALU_OUT_29 (1 BIT))
  Result47/1 -> Display47/1
  ALU_7/2(CARRY_OUT (1 BIT)) -> ALU_8/1(CARRY_IN (1 BIT))
  B_19/1 -> ALU_19/6(B_INPUT (1 BIT))
  ALU_43/2(CARRY_OUT (1 BIT)) -> ALU_44/1(CARRY_IN (1 BIT))
  B_28/1 -> ALU_28/6(B_INPUT (1 BIT))
  ALU_48/2(CARRY_OUT (1 BIT)) -> ALU_49/1(CARRY_IN (1 BIT))
  A_21/1 -> ALU_21/4(A_INPUT (1 BIT))
  ALU_39/2(CARRY_OUT (1 BIT)) -> ALU_40/1(CARRY_IN (1 BIT))
  A_41/1 -> ALU_41/4(A_INPUT (1 BIT))
  B_41/1 -> ALU_41/6(B_INPUT (1 BIT))
  B_35/1 -> ALU_35/6(B_INPUT (1 BIT))
  B_27/1 -> ALU_27/6(B_INPUT (1 BIT))
  A_56/1 -> ALU_56/4(A_INPUT (1 BIT))
  A_50/1 -> ALU_50/4(A_INPUT (1 BIT))
  Result40/1 -> Display40/1
  A_57/1 -> ALU_57/4(A_INPUT (1 BIT))
  ALU_41/2(CARRY_OUT (1 BIT)) -> ALU_42/1(CARRY_IN (1 BIT))
  Result51/1 -> Display51/1
  A_25/1 -> ALU_25/4(A_INPUT (1 BIT))
  Result46/1 -> Display46/1
  Result32/1 -> Display32/1
  B_60/1 -> ALU_60/6(B_INPUT (1 BIT))
  ALU_50/1(ALU_OUT (1 BIT)) -> Result51/1, ALU_OUT_32_BIT_1/19(ALU_OUT_18 (1 BIT)), ZERO/14
  A_42/1 -> ALU_42/4(A_INPUT (1 BIT))
  ALU_51/1(ALU_OUT (1 BIT)) -> Result50/1, ALU_OUT_32_BIT_1/20(ALU_OUT_19 (1 BIT)), ZERO/13
  ALU_30/1(ALU_OUT (1 BIT)) -> ZERO/34, Result31/1, ALU_OUT_32_BIT_00/31(ALU_OUT_30 (1 BIT))
  A_2/1 -> ALU_2/4(A_INPUT (1 BIT))
  ALU_37/2(CARRY_OUT (1 BIT)) -> ALU_38/1(CARRY_IN (1 BIT))
  ALU_58/2(CARRY_OUT (1 BIT)) -> ALU_59/1(CARRY_IN (1 BIT))
  Result38/1 -> Display38/1
  A_13/1 -> ALU_13/4(A_INPUT (1 BIT))
  A_14/1 -> ALU_14/4(A_INPUT (1 BIT))
  Result30/1 -> Display30/1
  B_24/1 -> ALU_24/6(B_INPUT (1 BIT))
  B_23/1 -> ALU_23/6(B_INPUT (1 BIT))
  B_12/1 -> ALU_12/6(B_INPUT (1 BIT))
  ALU_54/2(CARRY_OUT (1 BIT)) -> ALU_55/1(CARRY_IN (1 BIT))
  Result55/1 -> Display55/1
  Result52/1 -> Display52/1
  B_39/1 -> ALU_39/6(B_INPUT (1 BIT))
  B_26/1 -> ALU_26/6(B_INPUT (1 BIT))
  B_15/1 -> ALU_15/6(B_INPUT (1 BIT))
  B_22/1 -> ALU_22/6(B_INPUT (1 BIT))
  B_47/1 -> ALU_47/6(B_INPUT (1 BIT))
  A_28/1 -> ALU_28/4(A_INPUT (1 BIT))
  A_29/1 -> ALU_29/4(A_INPUT (1 BIT))
  B_30/1 -> ALU_30/6(B_INPUT (1 BIT))
  ALU_32/2(CARRY_OUT (1 BIT)) -> ALU_33/1(CARRY_IN (1 BIT))
  ALU_36/2(CARRY_OUT (1 BIT)) -> ALU_37/1(CARRY_IN (1 BIT))
  Result29/1 -> Display29/1
  A_24/1 -> ALU_24/4(A_INPUT (1 BIT))
  ALU_34/2(CARRY_OUT (1 BIT)) -> ALU_35/1(CARRY_IN (1 BIT))
  B_7/1 -> ALU_7/6(B_INPUT (1 BIT))
  ALU_35/2(CARRY_OUT (1 BIT)) -> ALU_36/1(CARRY_IN (1 BIT))
  A_18/1 -> ALU_18/4(A_INPUT (1 BIT))
  A_31/1 -> ALU_31/4(A_INPUT (1 BIT))
  Result39/1 -> Display39/1
  Result37/1 -> Display37/1
  ALU_14/2(CARRY_OUT (1 BIT)) -> ALU_15/1(CARRY_IN (1 BIT))
  A_51/1 -> ALU_51/4(A_INPUT (1 BIT))
  ALU_29/2(CARRY_OUT (1 BIT)) -> ALU_30/1(CARRY_IN (1 BIT))
  Result28/1 -> Display28/1
  B_11/1 -> ALU_11/6(B_INPUT (1 BIT))
  A_53/1 -> ALU_53/4(A_INPUT (1 BIT))
  A_1/1 -> ALU_1/4(A_INPUT (1 BIT))
  B_0/1 -> ALU_0/6(B_INPUT (1 BIT))
  Result27/1 -> Display27/1
  A_5/1 -> ALU_5/4(A_INPUT (1 BIT))
  ALU_26/2(CARRY_OUT (1 BIT)) -> ALU_27/1(CARRY_IN (1 BIT))
  A_59/1 -> ALU_59/4(A_INPUT (1 BIT))
  Result56/1 -> Display56/1
  A_46/1 -> ALU_46/4(A_INPUT (1 BIT))
  ALU_57/2(CARRY_OUT (1 BIT)) -> ALU_58/1(CARRY_IN (1 BIT))
  B_3/1 -> ALU_3/6(B_INPUT (1 BIT))
  ALU_63/2(CARRY_OUT (1 BIT)) -> Register2/1
  Result3/1 -> Display3/1
  ALU_2/2(CARRY_OUT (1 BIT)) -> ALU_3/1(CARRY_IN (1 BIT))
  A_7/1 -> ALU_7/4(A_INPUT (1 BIT))
  ALU_19/2(CARRY_OUT (1 BIT)) -> ALU_20/1(CARRY_IN (1 BIT))
  B_58/1 -> ALU_58/6(B_INPUT (1 BIT))
  B_63/1 -> ALU_63/6(B_INPUT (1 BIT))
  B_62/1 -> ALU_62/6(B_INPUT (1 BIT))
  ALU_62/2(CARRY_OUT (1 BIT)) -> ALU_63/1(CARRY_IN (1 BIT))
  B_36/1 -> ALU_36/6(B_INPUT (1 BIT))
  B_37/1 -> ALU_37/6(B_INPUT (1 BIT))
  B_5/1 -> ALU_5/6(B_INPUT (1 BIT))
  A_4/1 -> ALU_4/4(A_INPUT (1 BIT))
  B_9/1 -> ALU_9/6(B_INPUT (1 BIT))
  A_36/1 -> ALU_36/4(A_INPUT (1 BIT))
  B_16/1 -> ALU_16/6(B_INPUT (1 BIT))
  A_44/1 -> ALU_44/4(A_INPUT (1 BIT))
  B_45/1 -> ALU_45/6(B_INPUT (1 BIT))
  ALU_55/2(CARRY_OUT (1 BIT)) -> ALU_56/1(CARRY_IN (1 BIT))
  B_40/1 -> ALU_40/6(B_INPUT (1 BIT))
  ALU_OUT_32_BIT_00/1(ALU_OUT (32 BIT)) -> Concat1/2
  Register/1 -> ZERO (1 BIT)/1
  Register1/1 -> ALU_OUT (64 BIT)/1
  Register2/1 -> CARRY_OUT (1 BIT)/1
